simulink model "motor_model"  (R2022b)
settings: Solver=VariableStepAuto  StartTime=0.0  StopTime=0.5  MaxStep=1e-3  RelTol=1e-3
values from neighbouring files (symbols this model uses):
  lambda = 0.9995    [loadData.m]
  lamdVec = mot.Ld*idVec + mot.lammg    [loadData.m]
  lamqVec = mot.Lq*iqVec    [loadData.m]
undefined symbols (not defined in the file or in its folder): inv, mot, PI
libraries: simulink x9
settings Model: Creator=Utente  LastModifiedBy=luca.salviato
settings SolverCC: AlgebraicLoopSolver=TrustRegion
settings DebuggingCC: UnconnectedInputMsg=warning  UnconnectedOutputMsg=warning  UnconnectedLineMsg=warning  SFMachineParentedDataDiag=warning
settings ModelReferenceCC: EnableRefExpFcnMdlSchedulingChecks=on

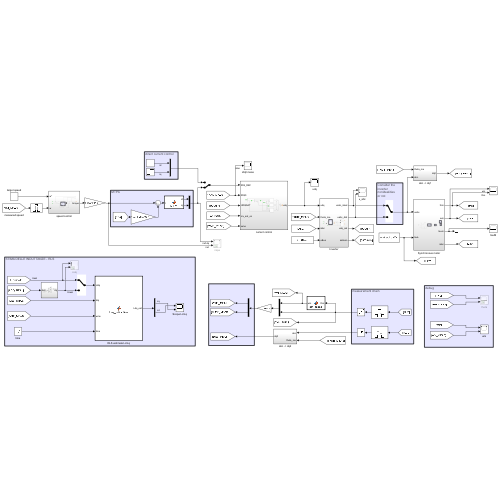
[thumbnail: Simulink's stored preview of the top-level diagram]
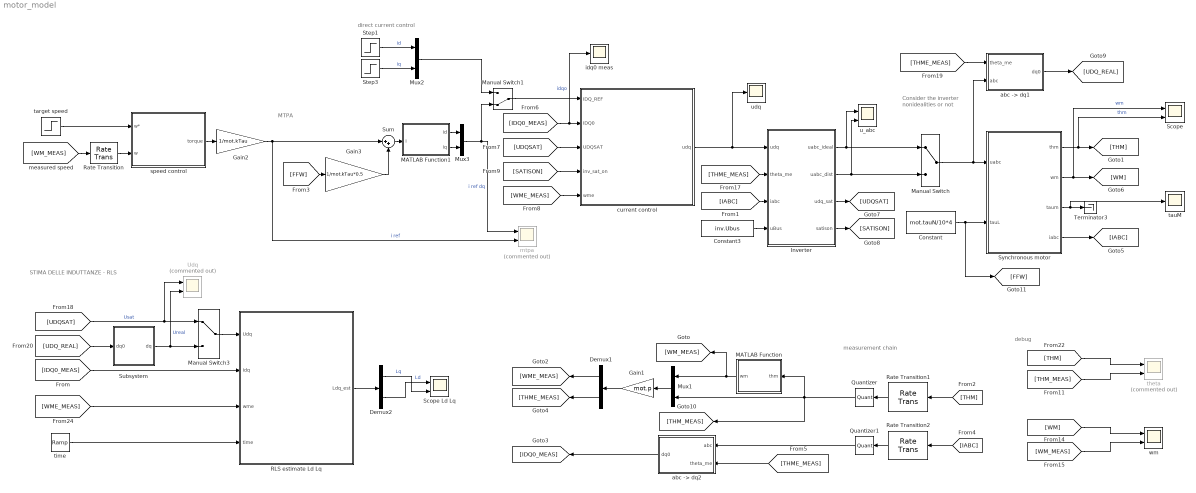
== system motor_model ==
  note: MTPA
  note: STIMA DELLE INDUTTANZE - RLS
  note: debug
  note: direct current control
  note: measurement chain
  note: Consider the
      | inverter
      | nonidealities
      | or not
  Constant : Constant  Value=mot.tauN/10*4
  Constant3 : Constant  Value=inv.Ubus
  Demux1 : Demux  Outputs=2
  Demux2 : Demux  Outputs=2
  Gain1 : Gain  Gain=mot.p
  Gain2 : Gain  Gain=1/mot.kTau
  Gain3 : Gain  Gain=1/mot.kTau*0.5
  Inverter : Subsystem
  MATLAB Function : MATLAB Function  TreatAsAtomicUnit=on
  MATLAB Function1 : MATLAB Function  TreatAsAtomicUnit=on
  Manual Switch : ManualSwitch
  Manual Switch1 : ManualSwitch  CurrentSetting=0
  Manual Switch3 : ManualSwitch
  Mux1 : Mux  Inputs=2
  Mux2 : Mux  Inputs=2
  Mux3 : Mux  Inputs=2
  Quantizer : Quantizer  QuantizationInterval=meas.enc.q
  Quantizer1 : Quantizer  QuantizationInterval=meas.cur.adc.q
  RLS estimate Ld Lq : MATLAB Function  TreatAsAtomicUnit=on
  Rate Transition : RateTransition  Deterministic=off  OutPortSampleTime=PI.vel.Ts
  Rate Transition1 : RateTransition  OutPortSampleTime=inv.Ts
  Rate Transition2 : RateTransition  Deterministic=off  OutPortSampleTime=inv.Ts
  Scope : Scope  NumInputPorts=2
  Scope Ld Lq : Scope  NumInputPorts=2
  Step1 : Step  Time=0.02  After=0.3  SampleTime=PI.vel.Ts
  Step3 : Step  Time=0.02  After=0  SampleTime=PI.vel.Ts
  Subsystem : Subsystem
  Sum : Sum  Inputs=|++
  Synchronous motor : Subsystem
  Terminator3 : Terminator
  Udq : Scope  Commented=on  NumInputPorts=2
  "abc -> dq1" : Subsystem
  "abc -> dq2" : Subsystem
  current control : Subsystem
  idq0 meas : Scope
  mtpa : Scope  Commented=on  NumInputPorts=2
  speed control : Subsystem
  target speed : Step  Time=0.02  After=50  SampleTime=PI.vel.Ts
  tauM : Scope
  theta : Scope  Commented=on  NumInputPorts=2
  time : simulink/Sources/Ramp  slope=1  start=0  InitialOutput=0  VectorParams1D=off
  u_abc : Scope  NumInputPorts=2
  udq : Scope
  wm : Scope  NumInputPorts=2
  wires:
  Synchronous motor/1(thm) -> Scope/2, [THM]  "thm"
  Synchronous motor/2(wm) -> Scope/1, [WM]  "wm"
  Synchronous motor/3(taum) -> tauM/1, Terminator3/1
  Synchronous motor/4(iabc) -> [IABC]
  Manual Switch/1 -> "abc -> dq1"/2(abc), Synchronous motor/1(uabc)
  [THME_MEAS] -> Inverter/2(theta_me)
  [IABC] -> Inverter/3(iabc)
  Constant3/1 -> Inverter/4(uBus)
  Inverter/1(uabc_ideal) -> u_abc/1, Manual Switch/1
  Inverter/2(uabc_dist) -> u_abc/2, Manual Switch/2
  Gain1/1 -> Demux1/1
  Demux1/2 -> [THME_MEAS]
  "abc -> dq2"/1(dq0) -> [IDQ0_MEAS]
  [THME_MEAS] -> "abc -> dq2"/1(theta_me)
  [IDQ0_MEAS] -> current control/2(IDQ0), idq0 meas/1  "idqo"
  Inverter/3(udq_sat) -> [UDQSAT]
  Inverter/4(satison) -> [SATISON]
  Step1/1 -> Mux2/1  "id"
  current control/1(udq) -> Inverter/1(udq), udq/1
  Mux2/1 -> Manual Switch1/1
  [UDQSAT] -> current control/3(UDQSAT)
  [SATISON] -> current control/4(inv_sat_on)
  Gain2/1 -> mtpa/2, Sum/1  "i ref"
  speed control/1(torque) -> Gain2/1
  [WM_MEAS] -> Rate Transition/1
  Rate Transition1/1 -> Quantizer/1
  Rate Transition2/1 -> Quantizer1/1
  Quantizer/1 -> Mux1/2, MATLAB Function/1(thm), [THM_MEAS]
  Quantizer1/1 -> "abc -> dq2"/2(abc)
  Mux1/1 -> Gain1/1
  MATLAB Function/1(wm) -> [WM_MEAS], Mux1/1
  Rate Transition/1 -> speed control/2(w)
  [THM] -> Rate Transition1/1
  [IABC] -> Rate Transition2/1
  [THM] -> theta/1
  [THM_MEAS] -> theta/2
  [WM] -> wm/1
  [WM_MEAS] -> wm/2
  [WME_MEAS] -> current control/5(wme)
  Demux1/1 -> [WME_MEAS]
  [UDQSAT] -> Manual Switch3/1, Udq/1  "Usat"
  [IDQ0_MEAS] -> RLS estimate Ld Lq/2(Idq)
  [WME_MEAS] -> RLS estimate Ld Lq/3(wme)
  RLS estimate Ld Lq/1(Ldq_est) -> Demux2/1
  MATLAB Function1/1(id) -> Mux3/1
  MATLAB Function1/2(iq) -> Mux3/2
  Mux3/1 -> mtpa/1, Manual Switch1/2  "i ref dq"
  Manual Switch1/1 -> current control/1(IDQ_REF)
  Demux2/1 -> Scope Ld Lq/2  "Lq"
  Demux2/2 -> Scope Ld Lq/1  "Ld"
  target speed/1 -> speed control/1(w*)
  Constant/1 -> Synchronous motor/2(tauL), [FFW]
  time/1 -> RLS estimate Ld Lq/4(time)
  Manual Switch3/1 -> RLS estimate Ld Lq/1(Udq)
  "abc -> dq1"/1(dq0) -> [UDQ_REAL]
  [THME_MEAS] -> "abc -> dq1"/1(theta_me)
  [UDQ_REAL] -> Subsystem/1(dq0)
  Subsystem/1(dq) -> Manual Switch3/2, Udq/2  "Ureal"
  Step3/1 -> Mux2/2  "iq"
  Sum/1 -> MATLAB Function1/1(I)
  Gain3/1 -> Sum/2
  [FFW] -> Gain3/1

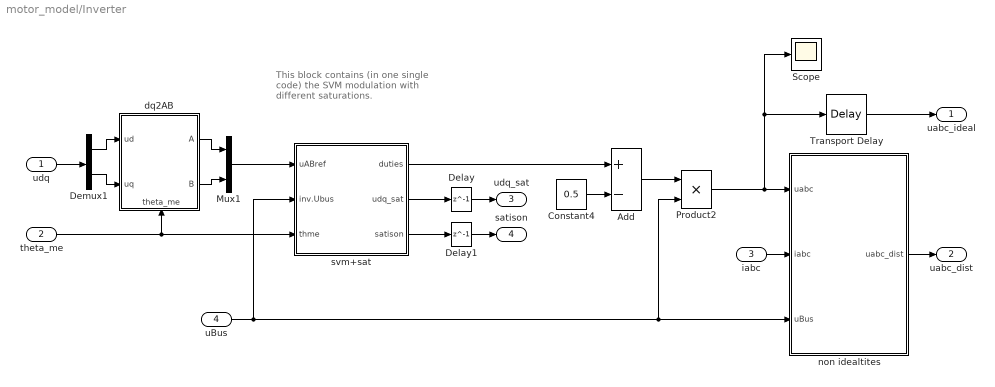
== system motor_model/Inverter ==
  note: This block contains (in one
      | single code) the SVM
      | modulation with different
      | saturations.
  udq : Inport
  theta_me : Inport  Port=2
  iabc : Inport  Port=3
  uBus : Inport  Port=4
  Add : Sum  Inputs=+-
  Constant4 : Constant  Value=0.5
  Delay : Delay  DelayLength=1  SampleTime=inv.Ts
  Delay1 : Delay  DelayLength=1  SampleTime=inv.Ts
  Demux1 : Demux  Outputs=2
  Mux1 : Mux  Inputs=2
  Product2 : Product
  Scope : Scope
  Transport Delay : TransportDelay  DelayTime=inv.Tpwm/2  BufferSize=10240
  dq2AB : Subsystem
      settings: PortSchema="{\"entries\":[{\"content\":{\"sides\":[{\"content\":{\"connectorIds\":[\"In1\",\"In2\"]},\"type\":\"ConnectorPlacement.EquallySpacedRectSide\",\"uuid\":\"508e90cc-8d20-4cd0-9210-55b91cc49af0\"},{\"content\":{\"connectorIds\":[\"Out1\",\"Out2\"],\"side\":\"RIGHT\"},\"type\":\"ConnectorPlacement.EquallySpacedRectSide\",\"uuid\":\"4bf96284-b8ec-4902-87e2-e0a0359215d2\"},{\"content\":{\"connectorIds\":[],\"side\":\"TOP\"},\"type\":\"ConnectorPlacement.EquallySpacedRectSide\",\"uuid\":\"d31ca5b0-df8f-443f-b3be-cff3e4b84ee6\"},{\"content\":{\"connectorIds\":[\"In3\"],\"side\":\"BOTTOM\"},\"type\":\"ConnectorPlacement.EquallySpacedRectSide\",\"uuid\":\"97c8cb02-9d30-416d-966b-7adbf36cdbfe\"}]},\"type\":\"ConnectorPlacement.EquallySpacedConnector\",\"uuid\":\"a4ed0bfe-09d9-422f-a69c-06bc783f2597\"}],\"packageUris\":[\"http://schema.mathworks.com/mf0/Connector/19700101\"],\"version\":\"1.0\"}"
  non idealtites : Subsystem
  svm+sat : Subsystem
  uabc_ideal : Outport
  uabc_dist : Outport  Port=2
  udq_sat : Outport  Port=3
  satison : Outport  Port=4
  wires:
  uBus/1 -> svm+sat/2(inv.Ubus), non idealtites/3(uBus), Product2/2
  Add/1 -> Product2/1
  dq2AB/1(A) -> Mux1/1
  svm+sat/1(duties) -> Add/1
  Constant4/1 -> Add/2
  dq2AB/2(B) -> Mux1/2
  udq/1 -> Demux1/1
  Mux1/1 -> svm+sat/1(uABref)
  Demux1/1 -> dq2AB/1(ud)
  Demux1/2 -> dq2AB/2(uq)
  theta_me/1 -> svm+sat/3(thme), dq2AB/3(theta_me)
  non idealtites/1(uabc_dist) -> uabc_dist/1
  iabc/1 -> non idealtites/2(iabc)
  Product2/1 -> Scope/1, Transport Delay/1, non idealtites/1(uabc)
  svm+sat/2(udq_sat) -> Delay/1
  svm+sat/3(satison) -> Delay1/1
  Transport Delay/1 -> uabc_ideal/1
  Delay1/1 -> satison/1
  Delay/1 -> udq_sat/1

== system motor_model/Subsystem ==
  dq0 : Inport
  Demux5 : Demux  Outputs=3
  Mux4 : Mux  Inputs=2
  Terminator1 : Terminator
  dq : Outport
  wires:
  Demux5/3 -> Terminator1/1
  Demux5/1 -> Mux4/1
  dq0/1 -> Demux5/1
  Demux5/2 -> Mux4/2
  Mux4/1 -> dq/1

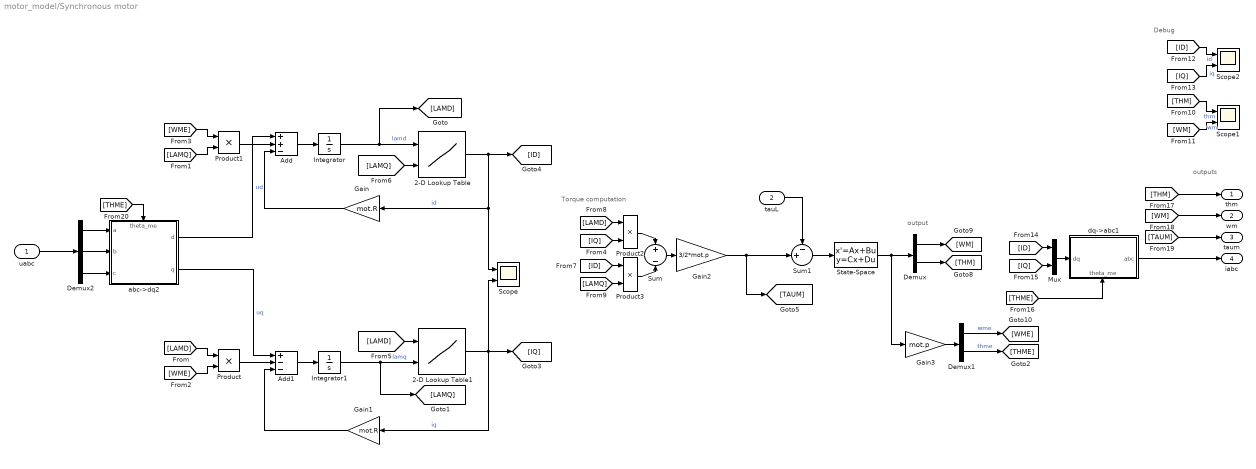
== system motor_model/Synchronous motor ==
  note: outputs
  note: Torque computation
  note: output
  note: Debug
  uabc : Inport
  tauL : Inport  Port=2
  2-D Lookup Table : Lookup_n-D  BreakpointsForDimension1=lamdVec  BreakpointsForDimension2=lamqVec  Table=idMap'  InternalRulePriority=Speed  RndMeth=Simplest
      settings: InputPortMap=u0,u1
  2-D Lookup Table1 : Lookup_n-D  BreakpointsForDimension1=lamdVec  BreakpointsForDimension2=lamqVec  Table=iqMap'  InternalRulePriority=Speed  RndMeth=Simplest
      settings: InputPortMap=u0,u1
  Add : Sum  Inputs=++-
  Add1 : Sum  Inputs=+--
  Demux : Demux  Outputs=2
  Demux1 : Demux  Outputs=2
  Demux2 : Demux  Outputs=3
  Gain : Gain  Gain=mot.R
  Gain1 : Gain  Gain=mot.R
  Gain2 : Gain  Gain=3/2*mot.p
  Gain3 : Gain  Gain=mot.p
  Integrator : Integrator  InitialCondition=mot.lammg
  Integrator1 : Integrator
  Mux : Mux  Inputs=2
  Product{,1..3} (4 alike) : Product
  Scope : Scope  NumInputPorts=2
  Scope1 : Scope  NumInputPorts=2
  Scope2 : Scope  NumInputPorts=2
  State-Space : StateSpace  A=[ -mot.B/mot.J 0 ; 1 0]  B=[1/mot.J ; 0]  C=eye(2)  D=[0; 0]  InitialCondition=[0;0]
  Sum : Sum  Inputs=+-
  Sum1 : Sum  Inputs=-+|
  abc->dq2 : Subsystem
      settings: PortSchema="{\"entries\":[{\"content\":{\"sides\":[{\"content\":{\"connectorIds\":[\"In1\",\"In2\",\"In3\"]},\"type\":\"ConnectorPlacement.EquallySpacedRectSide\",\"uuid\":\"fe8e17e5-51f9-4d76-9762-24844d5591a5\"},{\"content\":{\"connectorIds\":[\"Out1\",\"Out2\"],\"side\":\"RIGHT\"},\"type\":\"ConnectorPlacement.EquallySpacedRectSide\",\"uuid\":\"fe87c28e-6767-4170-9643-60ca24f3ac9b\"},{\"content\":{\"connectorIds\":[\"In4\"],\"side\":\"TOP\"},\"type\":\"ConnectorPlacement.EquallySpacedRectSide\",\"uuid\":\"dea0d24c-4fb3-4d95-8bb7-9e0d73dd5c70\"},{\"content\":{\"connectorIds\":[],\"side\":\"BOTTOM\"},\"type\":\"ConnectorPlacement.EquallySpacedRectSide\",\"uuid\":\"c69c3b56-495d-4db3-bf8e-d9a29d84b68b\"}]},\"type\":\"ConnectorPlacement.EquallySpacedConnector\",\"uuid\":\"884fba33-6802-455d-a170-b85a256a9851\"}],\"packageUris\":[\"http://schema.mathworks.com/mf0/Connector/19700101\"],\"version\":\"1.0\"}"
  dq->abc1 : Subsystem
      settings: PortSchema="{\"entries\":[{\"content\":{\"sides\":[{\"content\":{\"connectorIds\":[\"In1\"]},\"type\":\"ConnectorPlacement.EquallySpacedRectSide\",\"uuid\":\"4ffcad8d-ad4e-4b9f-9d99-70d9706481bd\"},{\"content\":{\"connectorIds\":[\"Out1\"],\"side\":\"RIGHT\"},\"type\":\"ConnectorPlacement.EquallySpacedRectSide\",\"uuid\":\"ca11e179-94fd-43b0-b2ab-d5b8ea31b40a\"},{\"content\":{\"connectorIds\":[],\"side\":\"TOP\"},\"type\":\"ConnectorPlacement.EquallySpacedRectSide\",\"uuid\":\"f9e7cc33-2dde-4aba-97f3-399a8c8ae3fe\"},{\"content\":{\"connectorIds\":[\"In2\"],\"side\":\"BOTTOM\"},\"type\":\"ConnectorPlacement.EquallySpacedRectSide\",\"uuid\":\"ae8b151b-7473-47fe-a384-ef12196a09bc\"}]},\"type\":\"ConnectorPlacement.EquallySpacedConnector\",\"uuid\":\"8c77ad63-71c2-4e35-a627-b120156b1a8b\"}],\"packageUris\":[\"http://schema.mathworks.com/mf0/Connector/R2020b\"],\"version\":\"1.0\"}"
  thm : Outport
  wm : Outport  Port=2
  taum : Outport  Port=3
  iabc : Outport  Port=4
  wires:
  abc->dq2/2(q) -> Add1/1  "uq"
  Demux1/1 -> [WME]  "wme"
  Sum1/1 -> State-Space/1
  Product3/1 -> Sum/2
  Gain1/1 -> Add1/3
  [THME] -> abc->dq2/4(theta_me)
  Gain/1 -> Add/3
  2-D Lookup Table1/1 -> Gain1/1, [IQ], Scope/2  "iq"
  Product/1 -> Add1/2
  Mux/1 -> dq->abc1/1(dq)
  [IQ] -> Product2/2
  Integrator1/1 -> 2-D Lookup Table1/2, [LAMQ]  "lamq"
  [ID] -> Product3/1
  Add1/1 -> Integrator1/1
  Integrator/1 -> 2-D Lookup Table/1, [LAMD]  "lamd"
  [IQ] -> Mux/2
  [LAMQ] -> 2-D Lookup Table/2
  [LAMD] -> Product/1
  Demux1/2 -> [THME]  "thme"
  [TAUM] -> taum/1
  [WM] -> wm/1
  Product1/1 -> Add/2
  Product2/1 -> Sum/1
  [LAMQ] -> Product1/2
  2-D Lookup Table/1 -> [ID], Scope/1, Gain/1  "id"
  Add/1 -> Integrator/1
  State-Space/1 -> Demux/1, Gain3/1
  [LAMD] -> 2-D Lookup Table1/1
  [THM] -> Scope1/1  "thm"
  [WME] -> Product1/1
  [WME] -> Product/2
  [THM] -> thm/1
  abc->dq2/1(d) -> Add/1  "ud"
  Demux2/2 -> abc->dq2/2(b)
  Sum/1 -> Gain2/1
  Demux2/1 -> abc->dq2/1(a)
  Gain2/1 -> Sum1/2, [TAUM]
  [IQ] -> Scope2/2  "iq"
  dq->abc1/1(abc) -> iabc/1
  [LAMQ] -> Product3/2
  [ID] -> Scope2/1  "id"
  [LAMD] -> Product2/1
  [THME] -> dq->abc1/2(theta_me)
  tauL/1 -> Sum1/1
  Demux/2 -> [THM]
  [ID] -> Mux/1
  Gain3/1 -> Demux1/1
  [WM] -> Scope1/2  "wm"
  Demux/1 -> [WM]
  uabc/1 -> Demux2/1
  Demux2/3 -> abc->dq2/3(c)

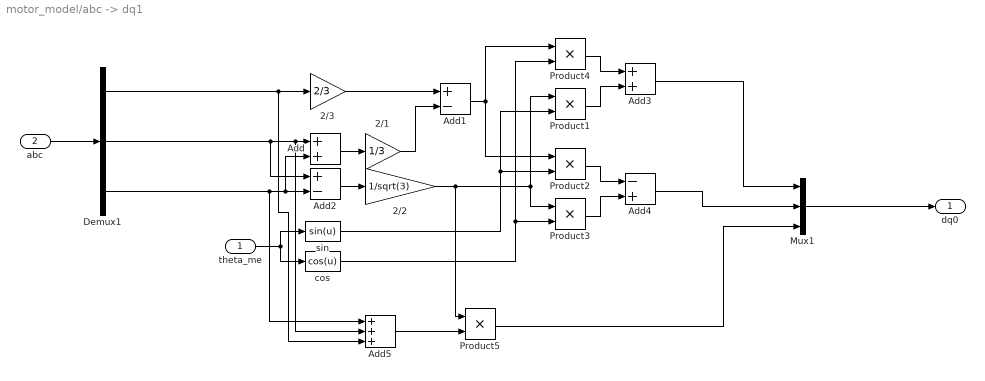
== system motor_model/abc -> dq1 ==
  theta_me : Inport
  abc : Inport  Port=2
  2/1 : Gain  Gain=1/3  SaturateOnIntegerOverflow=on  OutDataTypeStr=Inherit: Same as input  ParamDataTypeStr=Inherit: Same as input
  2/2 : Gain  Gain=1/sqrt(3)  SaturateOnIntegerOverflow=on  OutDataTypeStr=Inherit: Same as input  ParamDataTypeStr=Inherit: Same as input
  2/3 : Gain  Gain=2/3  SaturateOnIntegerOverflow=on  OutDataTypeStr=Inherit: Same as input  ParamDataTypeStr=Inherit: Same as input
  Add : Sum
  Add1 : Sum  Inputs=+-
  Add2 : Sum  Inputs=+-
  Add3 : Sum
  Add4 : Sum  Inputs=-+
  Add5 : Sum  Inputs=+++
  Demux1 : Demux  Outputs=3
  Mux1 : Mux  Inputs=3
  Product{1..5} (5 alike) : Product  RndMeth=Zero
  cos : Fcn  Expr=cos(u)
  sin : Fcn  Expr=sin(u)
  dq0 : Outport
  wires:
  abc/1 -> Demux1/1
  Mux1/1 -> dq0/1
  Product5/1 -> Mux1/3
  Add5/1 -> Product5/2
  Product3/1 -> Add4/2
  Product2/1 -> Add4/1
  Product1/1 -> Add3/2
  Product4/1 -> Add3/1
  Add4/1 -> Mux1/2
  Add3/1 -> Mux1/1
  sin/1 -> Product1/2, Product2/2
  2/2/1 -> Product1/1, Product3/1, Product5/1
  cos/1 -> Product4/2, Product3/2
  Add1/1 -> Product4/1, Product2/1
  theta_me/1 -> cos/1, sin/1
  Add/1 -> 2/1/1
  2/1/1 -> Add1/2
  Demux1/1 -> 2/3/1, Add5/3
  2/3/1 -> Add1/1
  Demux1/3 -> Add/2, Add2/2, Add5/1
  Add2/1 -> 2/2/1
  Demux1/2 -> Add/1, Add5/2, Add2/1

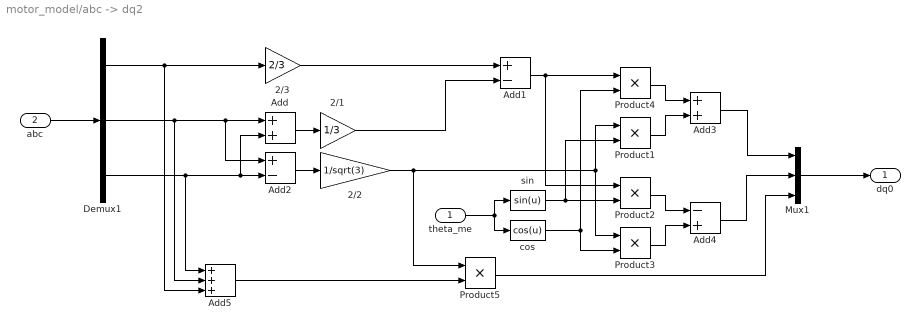
== system motor_model/abc -> dq2 ==
  theta_me : Inport
  abc : Inport  Port=2
  2/1 : Gain  Gain=1/3  SaturateOnIntegerOverflow=on  OutDataTypeStr=Inherit: Same as input  ParamDataTypeStr=Inherit: Same as input
  2/2 : Gain  Gain=1/sqrt(3)  SaturateOnIntegerOverflow=on  OutDataTypeStr=Inherit: Same as input  ParamDataTypeStr=Inherit: Same as input
  2/3 : Gain  Gain=2/3  SaturateOnIntegerOverflow=on  OutDataTypeStr=Inherit: Same as input  ParamDataTypeStr=Inherit: Same as input
  Add : Sum
  Add1 : Sum  Inputs=+-
  Add2 : Sum  Inputs=+-
  Add3 : Sum
  Add4 : Sum  Inputs=-+
  Add5 : Sum  Inputs=+++
  Demux1 : Demux  Outputs=3
  Mux1 : Mux  Inputs=3
  Product{1..5} (5 alike) : Product  RndMeth=Zero
  cos : Fcn  Expr=cos(u)
  sin : Fcn  Expr=sin(u)
  dq0 : Outport
  wires:
  Demux1/2 -> Add/1, Add2/1, Add5/2
  Add2/1 -> 2/2/1
  Demux1/3 -> Add/2, Add2/2, Add5/1
  2/3/1 -> Add1/1
  Demux1/1 -> Add5/3, 2/3/1
  2/1/1 -> Add1/2
  Add/1 -> 2/1/1
  theta_me/1 -> sin/1, cos/1
  Add1/1 -> Product4/1, Product2/1
  cos/1 -> Product3/2, Product4/2
  2/2/1 -> Product1/1, Product3/1, Product5/1
  sin/1 -> Product2/2, Product1/2
  Add3/1 -> Mux1/1
  Add4/1 -> Mux1/2
  Product4/1 -> Add3/1
  Product1/1 -> Add3/2
  Product2/1 -> Add4/1
  Product3/1 -> Add4/2
  Add5/1 -> Product5/2
  Product5/1 -> Mux1/3
  Mux1/1 -> dq0/1
  abc/1 -> Demux1/1

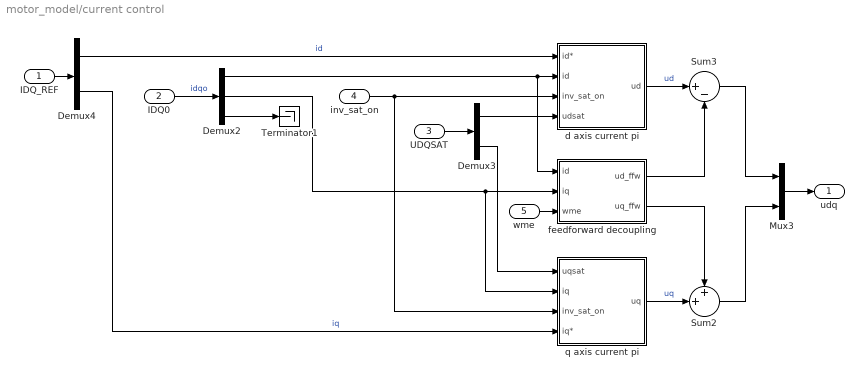
== system motor_model/current control ==
  IDQ_REF : Inport
  IDQ0 : Inport  Port=2
  UDQSAT : Inport  Port=3
  inv_sat_on : Inport  Port=4
  wme : Inport  Port=5
  Demux2 : Demux  Outputs=3
  Demux3 : Demux  Outputs=2
  Demux4 : Demux  Outputs=2
  Mux3 : Mux  Inputs=2
  Sum2 : Sum  Inputs=++|
  Sum3 : Sum  Inputs=|+-
  Terminator1 : Terminator
  d axis current pi : Subsystem
  feedforward decoupling : Subsystem
  q axis current pi : Subsystem
  udq : Outport
  wires:
  Demux3/1 -> d axis current pi/4(udsat)
  q axis current pi/1(uq) -> Sum2/2  "uq"
  Demux3/2 -> q axis current pi/1(uqsat)
  d axis current pi/1(ud) -> Sum3/1  "ud"
  Demux2/2 -> q axis current pi/2(iq), feedforward decoupling/2(iq)
  Demux4/2 -> q axis current pi/4(iq*)  "iq"
  Sum3/1 -> Mux3/1
  Sum2/1 -> Mux3/2
  inv_sat_on/1 -> d axis current pi/3(inv_sat_on), q axis current pi/3(inv_sat_on)
  Demux4/1 -> d axis current pi/1(id*)  "id"
  Mux3/1 -> udq/1
  feedforward decoupling/1(ud_ffw) -> Sum3/2
  feedforward decoupling/2(uq_ffw) -> Sum2/1
  UDQSAT/1 -> Demux3/1
  Demux2/1 -> feedforward decoupling/1(id), d axis current pi/2(id)
  IDQ_REF/1 -> Demux4/1
  wme/1 -> feedforward decoupling/3(wme)
  IDQ0/1 -> Demux2/1  "idqo"
  Demux2/3 -> Terminator1/1

== system motor_model/speed control ==
  note: euler forward integrator
  w* : Inport
  w : Inport  Port=2
  Delay : Delay  DelayLength=1  SampleTime=PI.vel.Ts
  Delay1 : Delay  DelayLength=1  SampleTime=PI.vel.Ts
  Gain3 : Gain  Gain=PI.vel.kp
  Gain4 : Gain  Gain=PI.vel.ki
  Gain5 : Gain  Gain=PI.vel.kt
  Saturation : Saturate  UpperLimit=mot.IN*mot.kTau  LowerLimit=-mot.IN*mot.kTau
  Scope : Scope  NumInputPorts=4
  Sum1 : Sum  Inputs=|+-
  Sum2 : Sum  Inputs=+-
  Sum3 : Sum  Inputs=|+-
  Sum4 : Sum  Inputs=|++
  Sum5 : Sum
  torque : Outport
  wires:
  Gain4/1 -> Sum1/1
  Sum3/1 -> Scope/1, Gain3/1, Gain4/1  "errore"
  Delay1/1 -> Sum5/2
  Sum4/1 -> Sum2/1, Saturation/1
  Sum5/1 -> Delay1/1, Sum4/2, Scope/3  "integrale"
  Gain3/1 -> Scope/2, Sum4/1  "propozionale"
  Saturation/1 -> Scope/4, torque/1, Sum2/2  "uscita in coppia"
  Gain5/1 -> Sum1/2
  Sum2/1 -> Gain5/1
  w/1 -> Sum3/2
  Delay/1 -> Sum5/1
  Sum1/1 -> Delay/1
  w*/1 -> Sum3/1

== system motor_model/Inverter/dq2AB ==
  ud : Inport
  uq : Inport  Port=2
  theta_me : Inport  Port=3
  Mux : Mux  Inputs=2
  dq->abc2 : Subsystem
      settings: PortSchema="{\"entries\":[{\"content\":{\"sides\":[{\"content\":{\"connectorIds\":[\"In1\"]},\"type\":\"ConnectorPlacement.EquallySpacedRectSide\",\"uuid\":\"4ffcad8d-ad4e-4b9f-9d99-70d9706481bd\"},{\"content\":{\"connectorIds\":[\"Out1\",\"Out2\"],\"side\":\"RIGHT\"},\"type\":\"ConnectorPlacement.EquallySpacedRectSide\",\"uuid\":\"ca11e179-94fd-43b0-b2ab-d5b8ea31b40a\"},{\"content\":{\"connectorIds\":[],\"side\":\"TOP\"},\"type\":\"ConnectorPlacement.EquallySpacedRectSide\",\"uuid\":\"f9e7cc33-2dde-4aba-97f3-399a8c8ae3fe\"},{\"content\":{\"connectorIds\":[\"In2\"],\"side\":\"BOTTOM\"},\"type\":\"ConnectorPlacement.EquallySpacedRectSide\",\"uuid\":\"ae8b151b-7473-47fe-a384-ef12196a09bc\"}]},\"type\":\"ConnectorPlacement.EquallySpacedConnector\",\"uuid\":\"8c77ad63-71c2-4e35-a627-b120156b1a8b\"}],\"packageUris\":[\"http://schema.mathworks.com/mf0/Connector/19700101\"],\"version\":\"1.0\"}"
  A : Outport
  B : Outport  Port=2
  wires:
  Mux/1 -> dq->abc2/1(dq)
  uq/1 -> Mux/2
  ud/1 -> Mux/1
  dq->abc2/2(B) -> B/1
  dq->abc2/1(A) -> A/1
  theta_me/1 -> dq->abc2/2(theta_me)

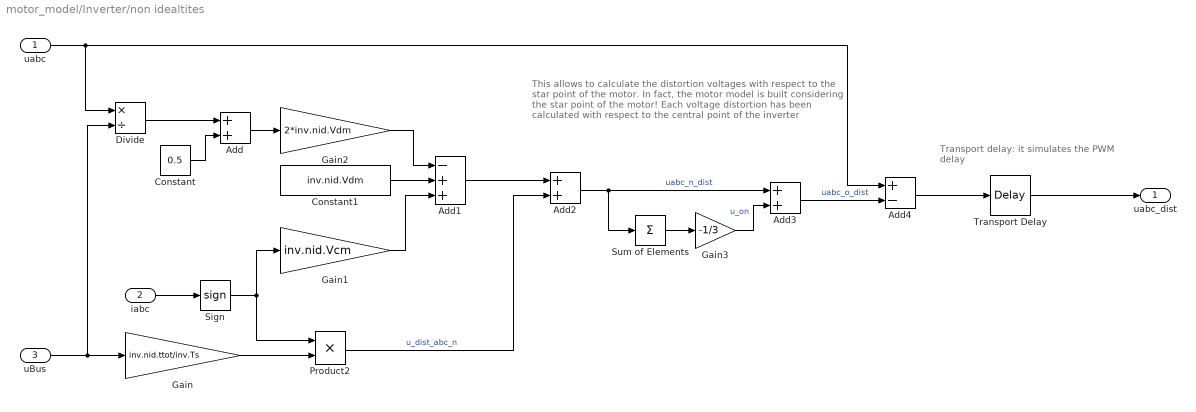
== system motor_model/Inverter/non idealtites ==
  note: Transport delay: it
      | simulates the PWM delay
  note: This allows to calculate the distortion voltages with
      | respect to the star point of the motor.
      | In fact, the motor model is built considering the
      | star point of the motor! Each voltage distortion
      | has been calculated with respect to the central
      | point of the inverter
  uabc : Inport
  iabc : Inport  Port=2
  uBus : Inport  Port=3
  Add : Sum
  Add1 : Sum  Inputs=-++
  Add2 : Sum
  Add3 : Sum
  Add4 : Sum  Inputs=+-
  Constant : Constant  Value=0.5
  Constant1 : Constant  Value=inv.nid.Vdm
  Divide : Product  Inputs=*/
  Gain : Gain  Gain=inv.nid.ttot/inv.Ts
  Gain1 : Gain  Gain=inv.nid.Vcm
  Gain2 : Gain  Gain=2*inv.nid.Vdm
  Gain3 : Gain  Gain=-1/3
  Product2 : Product
  Sign : Signum
  Sum of Elements : Sum  Inputs=+
  Transport Delay : TransportDelay  DelayTime=inv.Tpwm/2  BufferSize=10240
  uabc_dist : Outport
  wires:
  uBus/1 -> Divide/2, Gain/1
  Divide/1 -> Add/1
  Constant/1 -> Add/2
  iabc/1 -> Sign/1
  Sign/1 -> Product2/1, Gain1/1
  Gain/1 -> Product2/2
  Add/1 -> Gain2/1
  Gain2/1 -> Add1/1
  Constant1/1 -> Add1/2
  Gain1/1 -> Add1/3
  Product2/1 -> Add2/2  "u_dist_abc_n"
  Add1/1 -> Add2/1
  Add2/1 -> Add3/1, Sum of Elements/1  "uabc_n_dist"
  Sum of Elements/1 -> Gain3/1
  Gain3/1 -> Add3/2  "u_on"
  Add3/1 -> Add4/2  "uabc_o_dist"
  uabc/1 -> Divide/1, Add4/1
  Add4/1 -> Transport Delay/1
  Transport Delay/1 -> uabc_dist/1

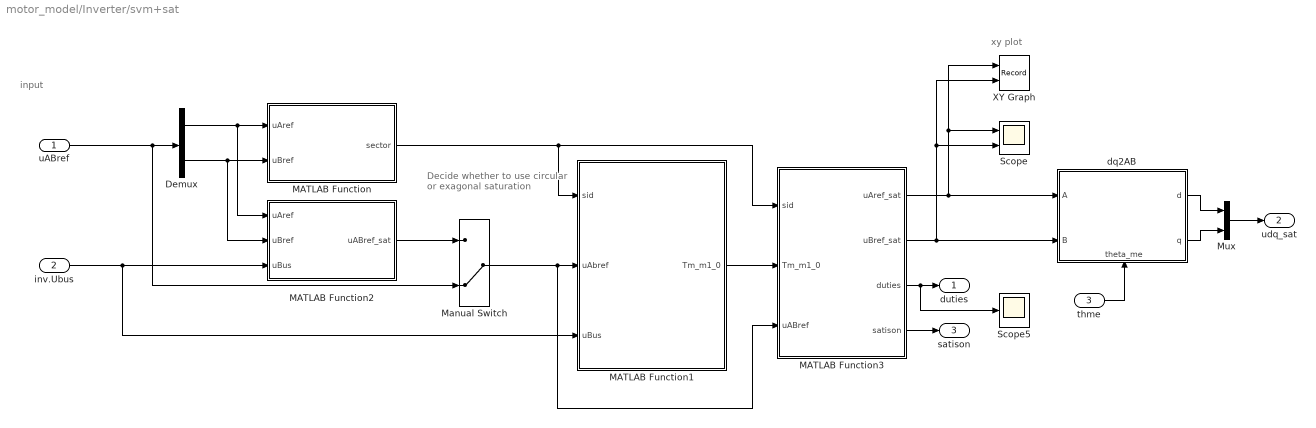
== system motor_model/Inverter/svm+sat ==
  note: xy plot
  note: Decide whether to
      | use circular or
      | exagonal saturation
  note: input
  uABref : Inport
  inv.Ubus : Inport  Port=2
  thme : Inport  Port=3
  Demux : Demux  Outputs=2
  MATLAB Function : MATLAB Function  TreatAsAtomicUnit=on
  MATLAB Function1 : MATLAB Function  TreatAsAtomicUnit=on
  MATLAB Function2 : MATLAB Function  TreatAsAtomicUnit=on
  MATLAB Function3 : MATLAB Function  TreatAsAtomicUnit=on
  Manual Switch : ManualSwitch  CurrentSetting=0
  Mux : Mux  Inputs=2
  Scope : Scope  NumInputPorts=2
  Scope5 : Scope
  XY Graph : Record  FileSettingsInternal="{\"entries\":[{\"content\":{\"excelSettings\":{\"content\":{},\"type\":\"Streamout.ExcelSettings\"}},\"type\":\"Streamout.FileSettingStorage\",\"uuid\":\"\"}],\"packageUris\":[\"http:\\/\\/schema.mathworks.com\\/mf0\\/streamout_blocks\\/R2020a\"],\"version\":\"1.0\"}"  Layout=[1 1]  SignalsInternal="{\"entries\":[{\"content\":{\"signals\":[{\"content\":{\"blockPath\":[],\"channel\":[],\"dimensions\":[1],\"domain\":\"\",\"lineColor\":\"#a2142f\",\"plots\":[1],\"port\":1,\"sid\":[],\"signalID\":568,\"signalName\":\"MATLAB Function3:1\"},\"type\":\"RecordBlkView.Signal\",\"uuid\":\"\"},{\"content\":{\"blockPath\":[],\"channel\":[],\"dimensions\":[1],\"domain\":\"\",\"lineColor\":\"#139fff\",\"plots\":[1],\"port\":2,\"sid\":[],\"signalID\":571,\"signalName\":\"MATLAB Function3:2\"},\"type\":\"RecordBlkView.Signal\",\"uuid\":\"\"}]},\"type\":\"RecordBlkView.InputSignals\",\"uuid\":\"\"}],\"packageUris\":[\"http:\\/\\/schema.mathworks.com\\/mf0\\/streamout_blocks\\/R2020a\"],\"version\":\"1.0\"}"  VisualizationBindings="{\"xyplotplugin\":{\"info\":[{\"series\":[{\"bindingParametersList\":[{\"parameter\":\"X-Axis\",\"signalID\":568,\"signalName\":\"MATLAB Function3:1\"},{\"parameter\":\"Y-Axis\",\"signalID\":571,\"signalName\":\"MATLAB Function3:2\"}],\"seriesID\":30743}],\"subplotID\":1}]}}"  CompatibilityTag=XY  st=-1
  dq2AB : Subsystem
      settings: PortSchema="{\"entries\":[{\"content\":{\"sides\":[{\"content\":{\"connectorIds\":[\"In1\",\"In2\"]},\"type\":\"ConnectorPlacement.EquallySpacedRectSide\",\"uuid\":\"508e90cc-8d20-4cd0-9210-55b91cc49af0\"},{\"content\":{\"connectorIds\":[\"Out1\",\"Out2\"],\"side\":\"RIGHT\"},\"type\":\"ConnectorPlacement.EquallySpacedRectSide\",\"uuid\":\"4bf96284-b8ec-4902-87e2-e0a0359215d2\"},{\"content\":{\"connectorIds\":[],\"side\":\"TOP\"},\"type\":\"ConnectorPlacement.EquallySpacedRectSide\",\"uuid\":\"d31ca5b0-df8f-443f-b3be-cff3e4b84ee6\"},{\"content\":{\"connectorIds\":[\"In3\"],\"side\":\"BOTTOM\"},\"type\":\"ConnectorPlacement.EquallySpacedRectSide\",\"uuid\":\"97c8cb02-9d30-416d-966b-7adbf36cdbfe\"}]},\"type\":\"ConnectorPlacement.EquallySpacedConnector\",\"uuid\":\"a4ed0bfe-09d9-422f-a69c-06bc783f2597\"}],\"packageUris\":[\"http://schema.mathworks.com/mf0/Connector/19700101\"],\"version\":\"1.0\"}"
  duties : Outport
  udq_sat : Outport  Port=2
  satison : Outport  Port=3
  wires:
  uABref/1 -> Manual Switch/2, Demux/1
  MATLAB Function3/3(duties) -> Scope5/1, duties/1
  MATLAB Function/1(sector) -> MATLAB Function3/1(sid), MATLAB Function1/1(sid)
  MATLAB Function2/1(uABref_sat) -> Manual Switch/1
  inv.Ubus/1 -> MATLAB Function1/3(uBus), MATLAB Function2/3(uBus)
  Manual Switch/1 -> MATLAB Function3/3(uABref), MATLAB Function1/2(uAbref)
  MATLAB Function3/1(uAref_sat) -> dq2AB/1(A), XY Graph/1, Scope/1
  MATLAB Function3/2(uBref_sat) -> XY Graph/2, Scope/2, dq2AB/2(B)
  Demux/1 -> MATLAB Function2/1(uAref), MATLAB Function/1(uAref)
  Demux/2 -> MATLAB Function2/2(uBref), MATLAB Function/2(uBref)
  MATLAB Function1/1(Tm_m1_0) -> MATLAB Function3/2(Tm_m1_0)
  thme/1 -> dq2AB/3(theta_me)
  dq2AB/1(d) -> Mux/1
  dq2AB/2(q) -> Mux/2
  Mux/1 -> udq_sat/1
  MATLAB Function3/4(satison) -> satison/1

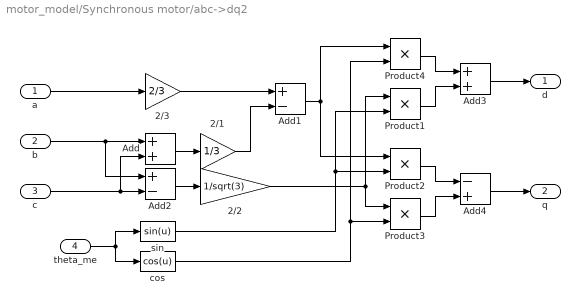
== system motor_model/Synchronous motor/abc->dq2 ==
  a : Inport
  b : Inport  Port=2
  c : Inport  Port=3
  theta_me : Inport  Port=4
  2/1 : Gain  Gain=1/3  SaturateOnIntegerOverflow=on  OutDataTypeStr=Inherit: Same as input  ParamDataTypeStr=Inherit: Same as input
  2/2 : Gain  Gain=1/sqrt(3)  SaturateOnIntegerOverflow=on  OutDataTypeStr=Inherit: Same as input  ParamDataTypeStr=Inherit: Same as input
  2/3 : Gain  Gain=2/3  SaturateOnIntegerOverflow=on  OutDataTypeStr=Inherit: Same as input  ParamDataTypeStr=Inherit: Same as input
  Add : Sum
  Add1 : Sum  Inputs=+-
  Add2 : Sum  Inputs=+-
  Add3 : Sum
  Add4 : Sum  Inputs=-+
  Product{1..4} (4 alike) : Product  RndMeth=Zero
  cos : Fcn  Expr=cos(u)
  sin : Fcn  Expr=sin(u)
  d : Outport
  q : Outport  Port=2
  wires:
  b/1 -> Add2/1, Add/1
  Add2/1 -> 2/2/1
  c/1 -> Add2/2, Add/2
  2/3/1 -> Add1/1
  a/1 -> 2/3/1
  2/1/1 -> Add1/2
  Add/1 -> 2/1/1
  theta_me/1 -> sin/1, cos/1
  Add1/1 -> Product2/1, Product4/1
  cos/1 -> Product3/2, Product4/2
  2/2/1 -> Product3/1, Product1/1
  sin/1 -> Product2/2, Product1/2
  Add3/1 -> d/1
  Add4/1 -> q/1
  Product4/1 -> Add3/1
  Product1/1 -> Add3/2
  Product2/1 -> Add4/1
  Product3/1 -> Add4/2

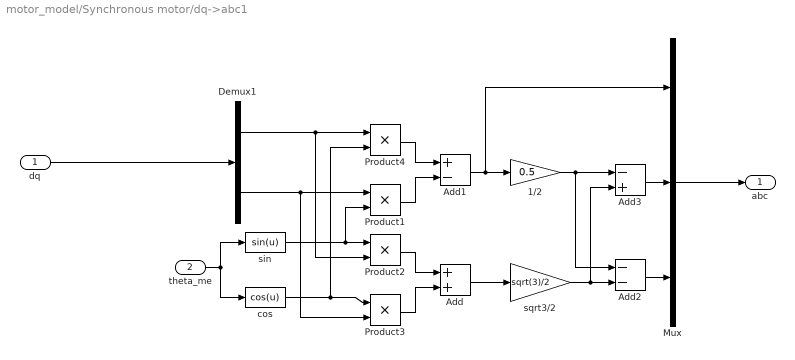
== system motor_model/Synchronous motor/dq->abc1 ==
  dq : Inport
  theta_me : Inport  Port=2
  1/2 : Gain  Gain=0.5  SaturateOnIntegerOverflow=on  OutDataTypeStr=Inherit: Same as input  ParamDataTypeStr=Inherit: Same as input
  Add : Sum
  Add1 : Sum  Inputs=+-
  Add2 : Sum  Inputs=--
  Add3 : Sum  Inputs=-+
  Demux1 : Demux  Outputs=2
  Mux : Mux  Inputs=3
  Product{1..4} (4 alike) : Product  RndMeth=Zero
  cos : Fcn  Expr=cos(u)
  sin : Fcn  Expr=sin(u)
  sqrt3/2 : Gain  Gain=sqrt(3)/2  SaturateOnIntegerOverflow=on  OutDataTypeStr=Inherit: Same as input  ParamDataTypeStr=Inherit: Same as input
  abc : Outport
  wires:
  theta_me/1 -> sin/1, cos/1
  Demux1/1 -> Product4/1, Product2/2
  cos/1 -> Product4/2, Product3/1
  Demux1/2 -> Product1/1, Product3/2
  sin/1 -> Product1/2, Product2/1
  Product4/1 -> Add1/1
  Product1/1 -> Add1/2
  Product2/1 -> Add/1
  Product3/1 -> Add/2
  Add1/1 -> 1/2/1, Mux/1
  Add/1 -> sqrt3/2/1
  1/2/1 -> Add3/1, Add2/1
  sqrt3/2/1 -> Add3/2, Add2/2
  Add3/1 -> Mux/2
  Add2/1 -> Mux/3
  dq/1 -> Demux1/1
  Mux/1 -> abc/1

== system motor_model/current control/d axis current pi ==
  note: euler forward
  id* : Inport
  id : Inport  Port=2
  inv_sat_on : Inport  Port=3
  udsat : Inport  Port=4
  Delay : Delay  DelayLength=1  SampleTime=PI.cur.Ts
  Delay1 : Delay  DelayLength=1  SampleTime=PI.cur.Ts
  Gain2 : Gain  Gain=PI.cur.kpd
  Gain3 : Gain  Gain=PI.cur.kid
  Sum : Sum  Inputs=|+-
  Sum1 : Sum
  Sum2 : Sum  Inputs=|++
  anti-windup : Subsystem
  ud : Outport
  wires:
  id*/1 -> Sum/1
  id/1 -> Sum/2
  Sum1/1 -> Sum2/2, Delay1/1
  Sum/1 -> anti-windup/1(e), Gain2/1  "error"
  Gain2/1 -> Sum2/1
  Sum2/1 -> ud/1  "ud"
  udsat/1 -> anti-windup/2(udsat)
  inv_sat_on/1 -> anti-windup/3(invsaton)
  anti-windup/1(anti_wu_out) -> Gain3/1
  Gain3/1 -> Delay/1
  Delay/1 -> Sum1/1
  Delay1/1 -> Sum1/2

== system motor_model/current control/feedforward decoupling ==
  id : Inport
  iq : Inport  Port=2
  wme : Inport  Port=3
  Gain2 : Gain  Gain=PI.cur.Lq
  Gain3 : Gain  Gain=PI.cur.Ld
  Gain4 : Gain  Gain=PI.cur.lammg
  Product : Product
  Product1 : Product
  Sum : Sum  Inputs=|++
  ud_ffw : Outport
  uq_ffw : Outport  Port=2
  wires:
  iq/1 -> Gain2/1
  Gain2/1 -> Product/1
  Gain3/1 -> Product1/2
  id/1 -> Gain3/1
  wme/1 -> Product1/1, Product/2, Gain4/1
  Sum/1 -> uq_ffw/1
  Product/1 -> ud_ffw/1
  Gain4/1 -> Sum/1
  Product1/1 -> Sum/2

== system motor_model/current control/q axis current pi ==
  note: euler forward
  uqsat : Inport
  iq : Inport  Port=2
  inv_sat_on : Inport  Port=3
  iq* : Inport  Port=4
  Delay2 : Delay  DelayLength=1  SampleTime=PI.cur.Ts
  Delay3 : Delay  DelayLength=1  SampleTime=PI.cur.Ts
  Gain2 : Gain  Gain=PI.cur.kpd
  Gain3 : Gain  Gain=PI.cur.kid
  Sum : Sum  Inputs=|+-
  Sum2 : Sum
  Sum5 : Sum  Inputs=|++
  anti-windup : Subsystem
  uq : Outport
  wires:
  inv_sat_on/1 -> anti-windup/3(invsaton)
  iq/1 -> Sum/2
  uqsat/1 -> anti-windup/2(uqsat)
  Sum5/1 -> uq/1  "uq"
  Delay3/1 -> Sum2/2
  Sum/1 -> anti-windup/1(e), Gain2/1  "error"
  Gain3/1 -> Delay2/1
  iq*/1 -> Sum/1
  Gain2/1 -> Sum5/1
  Delay2/1 -> Sum2/1
  Sum2/1 -> Sum5/2, Delay3/1
  anti-windup/1(anti_wu_out) -> Gain3/1

== system motor_model/Inverter/dq2AB/dq->abc2 ==
  dq : Inport
  theta_me : Inport  Port=2
  Add : Sum
  Add1 : Sum  Inputs=+-
  Demux1 : Demux  Outputs=2
  Product{1..4} (4 alike) : Product  RndMeth=Zero
  cos : Fcn  Expr=cos(u)
  sin : Fcn  Expr=sin(u)
  A : Outport
  B : Outport  Port=2
  wires:
  dq/1 -> Demux1/1
  Add/1 -> B/1  "B"
  Add1/1 -> A/1  "A"
  Product3/1 -> Add/2
  Product2/1 -> Add/1
  Product1/1 -> Add1/2
  Product4/1 -> Add1/1
  sin/1 -> Product2/1, Product1/2
  Demux1/2 -> Product3/2, Product1/1  "q"
  cos/1 -> Product3/1, Product4/2
  Demux1/1 -> Product2/2, Product4/1  "d"
  theta_me/1 -> cos/1, sin/1

== system motor_model/Inverter/svm+sat/dq2AB ==
  A : Inport
  B : Inport  Port=2
  theta_me : Inport  Port=3
  Mux : Mux  Inputs=2
  dq->abc2 : Subsystem
      settings: PortSchema="{\"entries\":[{\"content\":{\"sides\":[{\"content\":{\"connectorIds\":[\"In1\"]},\"type\":\"ConnectorPlacement.EquallySpacedRectSide\",\"uuid\":\"4ffcad8d-ad4e-4b9f-9d99-70d9706481bd\"},{\"content\":{\"connectorIds\":[\"Out1\",\"Out2\"],\"side\":\"RIGHT\"},\"type\":\"ConnectorPlacement.EquallySpacedRectSide\",\"uuid\":\"ca11e179-94fd-43b0-b2ab-d5b8ea31b40a\"},{\"content\":{\"connectorIds\":[],\"side\":\"TOP\"},\"type\":\"ConnectorPlacement.EquallySpacedRectSide\",\"uuid\":\"f9e7cc33-2dde-4aba-97f3-399a8c8ae3fe\"},{\"content\":{\"connectorIds\":[\"In2\"],\"side\":\"BOTTOM\"},\"type\":\"ConnectorPlacement.EquallySpacedRectSide\",\"uuid\":\"ae8b151b-7473-47fe-a384-ef12196a09bc\"}]},\"type\":\"ConnectorPlacement.EquallySpacedConnector\",\"uuid\":\"8c77ad63-71c2-4e35-a627-b120156b1a8b\"}],\"packageUris\":[\"http://schema.mathworks.com/mf0/Connector/19700101\"],\"version\":\"1.0\"}"
  d : Outport
  q : Outport  Port=2
  wires:
  Mux/1 -> dq->abc2/1(AB)
  B/1 -> Mux/2
  A/1 -> Mux/1
  dq->abc2/2(q) -> q/1
  dq->abc2/1(d) -> d/1
  theta_me/1 -> dq->abc2/2(theta_me)

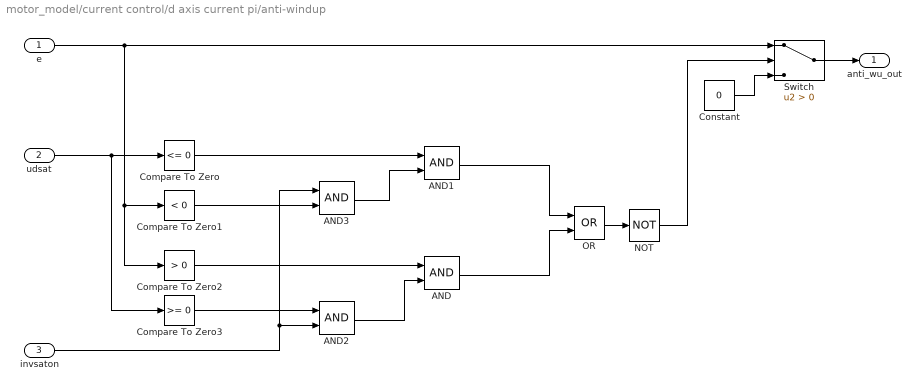
== system motor_model/current control/d axis current pi/anti-windup ==
  e : Inport
  udsat : Inport  Port=2
  invsaton : Inport  Port=3
  AND{,1..3} (4 alike) : Logic  AllPortsSameDT=off  OutDataTypeStr=boolean
  Compare To Zero : simulink/Logic and Bit Operations/Compare To Zero  relop=<=  OutDataTypeStr=boolean
  Compare To Zero1 : simulink/Logic and Bit Operations/Compare To Zero  relop=<  OutDataTypeStr=boolean
  Compare To Zero2 : simulink/Logic and Bit Operations/Compare To Zero  relop=>  OutDataTypeStr=boolean
  Compare To Zero3 : simulink/Logic and Bit Operations/Compare To Zero  relop=>=  OutDataTypeStr=boolean
  Constant : Constant  Value=0
  NOT : Logic  Operator=NOT  AllPortsSameDT=off  OutDataTypeStr=boolean
  OR : Logic  Operator=OR  AllPortsSameDT=off  OutDataTypeStr=boolean
  Switch : Switch  Criteria=u2 > Threshold  SaturateOnIntegerOverflow=off  InputSameDT=off
  anti_wu_out : Outport
  wires:
  NOT/1 -> Switch/2
  AND2/1 -> AND/2
  e/1 -> Compare To Zero1/1, Compare To Zero2/1, Switch/1
  AND/1 -> OR/2
  AND1/1 -> OR/1
  invsaton/1 -> AND3/1, AND2/2
  AND3/1 -> AND1/2
  OR/1 -> NOT/1
  Constant/1 -> Switch/3
  Compare To Zero/1 -> AND1/1
  Compare To Zero2/1 -> AND/1
  Compare To Zero3/1 -> AND2/1
  udsat/1 -> Compare To Zero3/1, Compare To Zero/1
  Compare To Zero1/1 -> AND3/2
  Switch/1 -> anti_wu_out/1

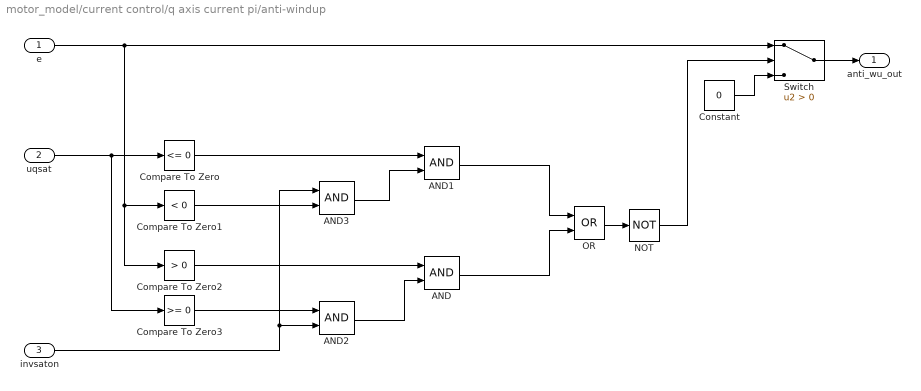
== system motor_model/current control/q axis current pi/anti-windup ==
  e : Inport
  uqsat : Inport  Port=2
  invsaton : Inport  Port=3
  AND{,1..3} (4 alike) : Logic  AllPortsSameDT=off  OutDataTypeStr=boolean
  Compare To Zero : simulink/Logic and Bit Operations/Compare To Zero  relop=<=  OutDataTypeStr=boolean
  Compare To Zero1 : simulink/Logic and Bit Operations/Compare To Zero  relop=<  OutDataTypeStr=boolean
  Compare To Zero2 : simulink/Logic and Bit Operations/Compare To Zero  relop=>  OutDataTypeStr=boolean
  Compare To Zero3 : simulink/Logic and Bit Operations/Compare To Zero  relop=>=  OutDataTypeStr=boolean
  Constant : Constant  Value=0
  NOT : Logic  Operator=NOT  AllPortsSameDT=off  OutDataTypeStr=boolean
  OR : Logic  Operator=OR  AllPortsSameDT=off  OutDataTypeStr=boolean
  Switch : Switch  Criteria=u2 > Threshold  SaturateOnIntegerOverflow=off  InputSameDT=off
  anti_wu_out : Outport
  wires:
  NOT/1 -> Switch/2
  AND2/1 -> AND/2
  e/1 -> Compare To Zero1/1, Compare To Zero2/1, Switch/1
  AND/1 -> OR/2
  AND1/1 -> OR/1
  invsaton/1 -> AND3/1, AND2/2
  AND3/1 -> AND1/2
  OR/1 -> NOT/1
  Constant/1 -> Switch/3
  Compare To Zero/1 -> AND1/1
  Compare To Zero2/1 -> AND/1
  Compare To Zero3/1 -> AND2/1
  uqsat/1 -> Compare To Zero3/1, Compare To Zero/1
  Compare To Zero1/1 -> AND3/2
  Switch/1 -> anti_wu_out/1

== system motor_model/Inverter/svm+sat/dq2AB/dq->abc2 ==
  AB : Inport
  theta_me : Inport  Port=2
  Add : Sum  Inputs=-+
  Add1 : Sum
  Demux1 : Demux  Outputs=2
  Product{1..4} (4 alike) : Product  RndMeth=Zero
  cos : Fcn  Expr=cos(u)
  sin : Fcn  Expr=sin(u)
  d : Outport
  q : Outport  Port=2
  wires:
  AB/1 -> Demux1/1
  Add/1 -> q/1
  Add1/1 -> d/1
  Product3/1 -> Add/2
  Product2/1 -> Add/1
  Product1/1 -> Add1/2
  Product4/1 -> Add1/1
  sin/1 -> Product2/1, Product1/2
  Demux1/2 -> Product3/2, Product1/1  "q"
  cos/1 -> Product3/1, Product4/2
  Demux1/1 -> Product2/2, Product4/1  "d"
  theta_me/1 -> cos/1, sin/1

== matlab function motor_model/Inverter/svm+sat/MATLAB Function1 ==
  data: sid input; Tm_m1_0 output; uAbref input; uBus input; inv parameter
function Tm_m1_0 = application_time(sid, uAbref, uBus, inv)
Tm_m1_0 = [0 ;0 ;0];
ua=uAbref(1);
ub=uAbref(2);

c=sqrt(3)*inv.Tpwm/inv.Ubus;
Tm_m1_0(1) = c*( ua*sin(sid*pi/3) - ub*cos(sid*pi/3) );
Tm_m1_0(2) = c*( -ua*sin((sid-1)*pi/3) + ub*cos((sid-1)*pi/3) );
Tm_m1_0(3) = inv.Tpwm - Tm_m1_0(1) - Tm_m1_0(2);

== matlab function motor_model/Inverter/svm+sat/MATLAB Function ==
  data: sector output; uAref input; uBref input
function sector = sector_identifier(uAref,uBref)

ua=uAref;
ub=uBref;

if(ub > 0) 
    if(abs(ua) > abs(ub)/sqrt(3))
        if (ua > 0)
            sector=1;
        else
            sector=3;
        end
    else
        sector=2;
    end
else
    if(abs(ua) > abs(ub)/sqrt(3))
        if (ua > 0)
            sector=6;
        else 
            sector=4;
        end
    else
        sector=5;
    end
end

== matlab function motor_model/Inverter/svm+sat/MATLAB Function2 ==
  data: uAref input; uBref input; uABref_sat output; uBus input
function uABref_sat = circle_sat( uAref,uBref, uBus)
ua = uAref;
ub=uBref;

uABref_sat = [ua ; ub];

modulo2 = ua^2 +ub^2;
if( modulo2 >= (uBus^2)/3 )
    k=sqrt( (uBus^2)/(3*modulo2) );
    uABref_sat(1) = ua*k;
    uABref_sat(2) = ub*k;
end

== matlab function motor_model/Inverter/svm+sat/MATLAB Function3 ==
  data: sid input; uAref_sat output; Tm_m1_0 input size=3; uABref input; uBref_sat output; duties output; inv parameter; satison output
function [uAref_sat, uBref_sat, duties, satison] = hexagonal_sat(sid, Tm_m1_0, uABref, inv)
duties=zeros(3,1);

if(Tm_m1_0(3) < 0)
    k=inv.Tpwm/( Tm_m1_0(1) + Tm_m1_0(2) );
    
    Tm_m1_0(1) = k*Tm_m1_0(1);
    Tm_m1_0(2) = k*Tm_m1_0(2);
    Tm_m1_0(3)=0;
    
    c=sqrt(3)*inv.Tpwm/inv.Ubus;
    uAB=[0;0];
    uAB= 1/c.*([ sin(sid*pi/3),-cos(sid*pi/3);
        -sin((sid-1)*pi/3), cos((sid-1)*pi/3) ])^(-1)*[Tm_m1_0(1);Tm_m1_0(2)];
    
    uAref_sat = uAB(1);
    uBref_sat = uAB(2);
    satison=1;
else
    uAref_sat = uABref(1);
    uBref_sat = uABref(2);
    satison=0;
end

switch (sid)
    case 1
        duties(1) = (Tm_m1_0(1)+Tm_m1_0(2)+Tm_m1_0(3)/2);
        duties(2) = (Tm_m1_0(2)+Tm_m1_0(3)/2);
        duties(3) = (Tm_m1_0(3)/2);
    case 2
        duties(1) = (Tm_m1_0(1)+Tm_m1_0(3)/2);
        duties(2) = (Tm_m1_0(1)+Tm_m1_0(2)+Tm_m1_0(3)/2);
        duties(3) = (Tm_m1_0(3)/2);
    case 3
        duties(2) = (Tm_m1_0(1)+Tm_m1_0(2)+Tm_m1_0(3)/2);
        duties(3) = (Tm_m1_0(2)+Tm_m1_0(3)/2);
        duties(1) = (Tm_m1_0(3)/2);
    case 4
        duties(3) = (Tm_m1_0(1)+Tm_m1_0(2)+Tm_m1_0(3)/2);
        duties(2) = (Tm_m1_0(1)+Tm_m1_0(3)/2);
        duties(1) = (Tm_m1_0(3)/2);
    case 5
        duties(3) = (Tm_m1_0(1)+Tm_m1_0(2)+Tm_m1_0(3)/2);
        duties(1) = (Tm_m1_0(2)+Tm_m1_0(3)/2);
        duties(2) = (Tm_m1_0(3)/2);
    case 6
        duties(1) = (Tm_m1_0(1)+Tm_m1_0(2)+Tm_m1_0(3)/2);
        duties(3) = (Tm_m1_0(1)+Tm_m1_0(3)/2);
        duties(2) = (Tm_m1_0(3)/2);
end
duties = duties./inv.Tpwm;

== matlab function motor_model/MATLAB Function ==
  data: thm input; wm output; meas parameter
function wm = get_speed(thm, meas) 
%TO DO: transform this script into a simple simulink transfer function
persistent buffer_thm

if isempty (buffer_thm)
    buffer_thm = zeros (1,meas.enc.nTabs);
end

wm = (thm - buffer_thm(meas.enc.nTabs)) / (meas.enc.nTabs*meas.enc.Ts);

for i = meas.enc.nTabs : -1 : 2
    buffer_thm(i) = buffer_thm(i-1);
end
buffer_thm(1) = thm;

== matlab function motor_model/MATLAB Function1 ==
  data: I input; id output; mot parameter; iq output
function [id,iq] = MTPA(I, mot)
if (I>0)
    id = (mot.lammg - sqrt(mot.lammg^2 + 8*((mot.Ld- mot.Lq)^2)*I^2))/(-4*(mot.Ld- mot.Lq) );
    iq = sqrt(I^2-id^2);
else
    id = (+mot.lammg - sqrt(mot.lammg^2 + 8*((mot.Ld- mot.Lq)^2)*I^2))/(-4*(mot.Ld- mot.Lq) );
    iq = -sqrt(I^2-id^2);
end

== matlab function motor_model/RLS estimate Ld Lq ==
  settings: updateMethod=DISCRETE
  data: Udq input; Ldq_est output size=2; Idq input; mot parameter; wme input; lambda parameter; time input
function Ldq_est = Ldq_estimation(Udq, Idq, mot, wme, lambda, time)
persistent Ldq_prec P_prec;

Rm=mot.R;
lammg=mot.lammg;

if isempty (P_prec)
    P_prec = diag([1,2])*100;
    Ldq_prec = [mot.Lq*1.3 ; mot.Ld*1.3];
end

if(time>0.2)
    y = [ Udq(2) - Rm*Idq(2) - lammg*wme
          Udq(1) - Rm*Idq(1) ];
    phi = [0   wme*Idq(1)
          -wme*Idq(2)  0]';
    K = P_prec*phi*inv( lambda.*eye(2) + phi'*P_prec*phi );
    P = ( eye(2)-K*phi' )*P_prec./lambda;
    err = y - phi'*Ldq_prec ;
    Ldq_est = Ldq_prec + K*err ;

    Ldq_prec = Ldq_est;
    P_prec = P;
else
    Ldq_est=Ldq_prec;
end
